simulink model "heli_quanser_base_D"  (R2025a)
settings: Solver=FixedStepAuto  StartTime=0.0  StopTime=30  FixedStep=0.001  RelTol=1e-3  EnableMultiTasking=on
values from neighbouring files (symbols this model uses):
  Ts = 1    [heli_ls_ident.m]    (also in minimos_cuadrados.m)
undefined symbols (not defined in the file or in its folder): B_p, B_y, g, J_eq_p, J_eq_y, K_pp, K_py, K_yp, K_yy, l_cm, m_heli, theta_0, VMAX_UPM_P, VMAX_UPM_Y
libraries: simulink x2, simulink_extras x1
settings Model: Creator=Jorge Romero  LastModifiedBy=Salvador
settings SolverCC: AlgebraicLoopSolver=TrustRegion
settings DataIOCC: LimitDataPoints=on  SaveFormat=Array  ReturnWorkspaceOutputs=off
settings OptimizationCC: ExpressionDepthLimit=2147483647.0  LifeSpan=inf
settings DebuggingCC: UnderspecifiedInitializationDetection=Classic  MergeDetectMultiDrivingBlocksExec=none  SolverPrmCheckMsg=warning  UnconnectedInputMsg=warning  UnconnectedOutputMsg=warning  UnconnectedLineMsg=warning  StateNameClashWarn=warning  SFUnexpectedBacktrackingDiag=warning  SFNoUnconditionalDefaultTransitionDiag=warning  SFExecutionAtInitializationDiag=none  ArithmeticOperatorsInVariantConditions=warning
settings HardwareCC: ProdBitPerPointer=32.0  ProdBitPerSizeT=32.0  ProdBitPerPtrDiffT=32.0  ProdLargestAtomicFloat=None  ProdIntDivRoundTo=Undefined  ProdEndianess=Unspecified  ProdWordSize=32.0  ProdHWDeviceType=32-bit Generic
settings ModelReferenceCC: EnableRefExpFcnMdlSchedulingChecks=on  PropagateSignalLabelsOutOfModel=off
settings SFSimCC: SimUseLocalCustomCode=off  CustomCodeUndefinedFunction=UseInterfaceOnly
settings RTWCC: RTWUseLocalCustomCode=off  GPUComputeCapability=3.5  DLArmComputeVersion=19.05
settings CodeAppCC: StateflowObjectComments=on
settings GRTTargetCC: TargetLangStandard=C89/C90 (ANSI)
settings ConfigComp: CovMetricSettings=dw  CovSaveCumulativeToWorkspaceVar=on  CovSaveSingleToWorkspaceVar=on  CovExternalEMLEnable=off

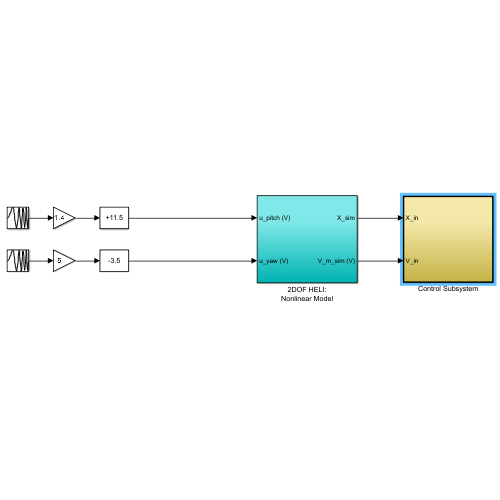
[thumbnail: Simulink's stored preview of the top-level diagram]
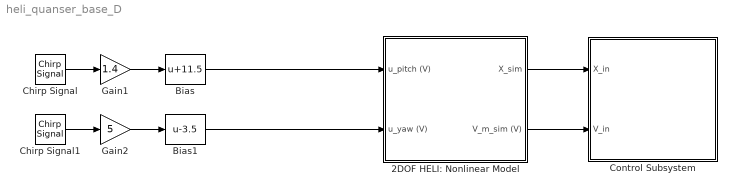
== system heli_quanser_base_D ==
  2DOF HELI: Nonlinear Model : Subsystem
  Bias : Bias  Bias=11.5  SaturateOnIntegerOverflow=off
  Bias1 : Bias  Bias=-3.5  SaturateOnIntegerOverflow=off
  Chirp Signal : simulink/Sources/Chirp Signal  f1=0.08  T=10  f2=1
  Chirp Signal1 : simulink/Sources/Chirp Signal  f1=0.05  T=100  f2=1
  Control Subsystem : Subsystem  TreatAsAtomicUnit=on
  Gain1 : Gain  Gain=1.4
  Gain2 : Gain  Gain=5
  wires:
  Gain2/1 -> Bias1/1
  Gain1/1 -> Bias/1
  Chirp Signal1/1 -> Gain2/1
  Chirp Signal/1 -> Gain1/1
  Bias/1 -> 2DOF HELI: Nonlinear Model/1(u_pitch (V))
  Bias1/1 -> 2DOF HELI: Nonlinear Model/2(u_yaw (V))
  2DOF HELI: Nonlinear Model/1(X_sim) -> Control Subsystem/1(X_in)
  2DOF HELI: Nonlinear Model/2(V_m_sim (V)) -> Control Subsystem/2(V_in)

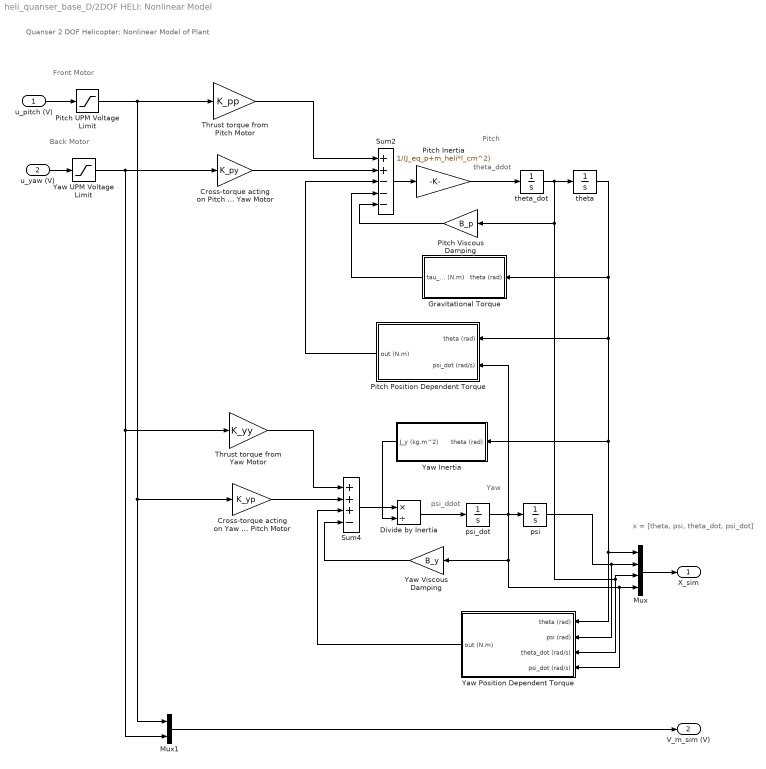
== system heli_quanser_base_D/2DOF HELI: Nonlinear Model ==
  note: Back Motor
  note: Front Motor
  note: x = [theta, psi, theta_dot, psi_dot]
  note: Quanser 2 DOF Helicopter: Nonlinear Model of Plant
  note: theta_ddot
  note: psi_ddot
  note: Pitch
  note: Yaw
  u_pitch (V) : Inport
  u_yaw (V) : Inport  Port=2
  Cross-torque acting on Pitch from Yaw Motor : Gain  Gain=K_py
  Cross-torque acting on Yaw from Pitch Motor : Gain  Gain=K_yp
  Divide by Inertia : Product  Inputs=*/
  Gravitational Torque : Subsystem
  Mux : Mux
  Mux1 : Mux  Inputs=2
  Pitch Inertia : Gain  Gain=1/(J_eq_p+m_heli*l_cm^2)
  Pitch Position Dependent Torque : Subsystem  AncestorBlock=heli_2d_lib/2DOF Helicopter: Nonlinear Model/Yaw Nonlinear Element
  Pitch UPM Voltage Limit : Saturate  UpperLimit=VMAX_UPM_P  LowerLimit=- VMAX_UPM_P
  Pitch Viscous Damping : Gain  Gain=B_p
  Sum2 : Sum  Inputs=++---
  Sum4 : Sum  Inputs=+++-
  Thrust torque from Pitch Motor : Gain  Gain=K_pp
  Thrust torque from Yaw Motor : Gain  Gain=K_yy
  Yaw Inertia : Subsystem
  Yaw Position Dependent Torque : Subsystem
  Yaw UPM Voltage Limit : Saturate  UpperLimit=VMAX_UPM_Y  LowerLimit=- VMAX_UPM_Y
  Yaw Viscous Damping : Gain  Gain=B_y
  psi : Integrator
  psi_dot : Integrator
  theta : Integrator  InitialCondition=theta_0  LimitOutput=on  UpperSaturationLimit=40.5*pi/180  LowerSaturationLimit=-40.5*pi/180
  theta_dot : Integrator
  X_sim : Outport
  V_m_sim (V) : Outport  Port=2
  wires:
  Pitch Position Dependent Torque/1(out (N.m)) -> Sum2/3
  Gravitational Torque/1(tau_g (N.m)) -> Sum2/4
  Pitch Viscous Damping/1 -> Sum2/5
  Cross-torque acting on Pitch from Yaw Motor/1 -> Sum2/2
  Thrust torque from Pitch Motor/1 -> Sum2/1
  Yaw Inertia/1(J_y (kg.m^2)) -> Divide by Inertia/2
  Divide by Inertia/1 -> psi_dot/1
  Sum4/1 -> Divide by Inertia/1
  Yaw Position Dependent Torque/1(out (N.m)) -> Sum4/3
  Yaw Viscous Damping/1 -> Sum4/4
  psi/1 -> Yaw Position Dependent Torque/2(psi (rad)), Mux/2
  Mux1/1 -> V_m_sim (V)/1
  Yaw UPM Voltage Limit/1 -> Thrust torque from Yaw Motor/1, Mux1/2, Cross-torque acting on Pitch from Yaw Motor/1
  Pitch UPM Voltage Limit/1 -> Mux1/1, Cross-torque acting on Yaw from Pitch Motor/1, Thrust torque from Pitch Motor/1
  Mux/1 -> X_sim/1
  theta/1 -> Gravitational Torque/1(theta (rad)), Pitch Position Dependent Torque/1(theta (rad)), Yaw Position Dependent Torque/1(theta (rad)), Mux/1, Yaw Inertia/1(theta (rad))
  Sum2/1 -> Pitch Inertia/1
  Pitch Inertia/1 -> theta_dot/1
  theta_dot/1 -> Pitch Viscous Damping/1, Yaw Position Dependent Torque/3(theta_dot (rad/s)), Mux/3, theta/1
  Thrust torque from Yaw Motor/1 -> Sum4/1
  Cross-torque acting on Yaw from Pitch Motor/1 -> Sum4/2
  psi_dot/1 -> Yaw Viscous Damping/1, Yaw Position Dependent Torque/4(psi_dot (rad/s)), Mux/4, Pitch Position Dependent Torque/2(psi_dot (rad/s)), psi/1
  u_pitch (V)/1 -> Pitch UPM Voltage Limit/1
  u_yaw (V)/1 -> Yaw UPM Voltage Limit/1

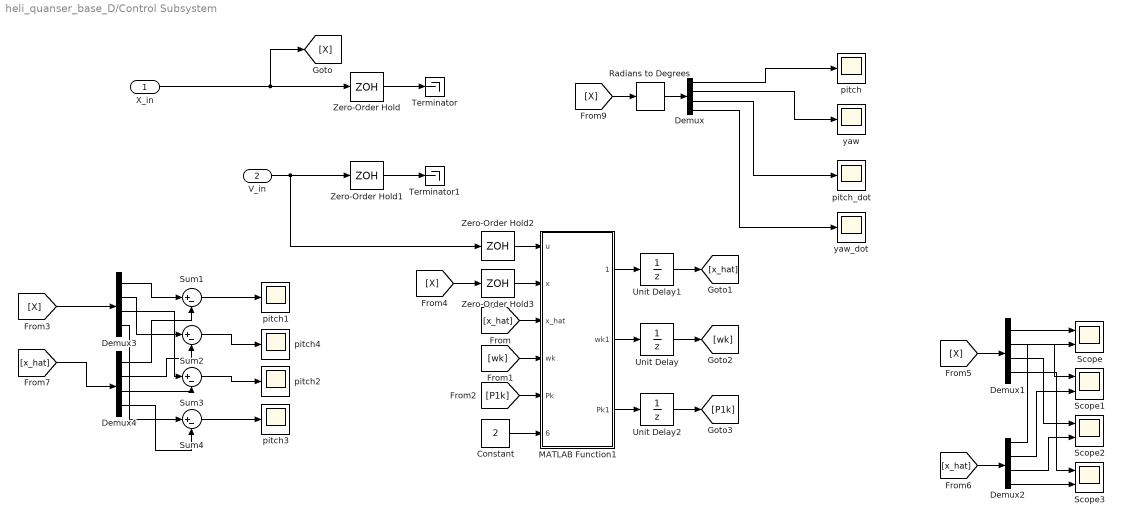
== system heli_quanser_base_D/Control Subsystem ==
  X_in : Inport
  V_in : Inport  Port=2
  Constant : Constant  Value=2
  Demux{,1..4} (5 alike) : Demux
      Demux settings: DisplayOption=none
  MATLAB Function1 : MATLAB Function  TreatAsAtomicUnit=on
  Radians to Degrees : simulink_extras/Transformations/Radians to Degrees
  Scope{,1..3} (4 alike) : Scope  NumInputPorts=2
      Scope settings: ActiveDisplayYMinimum=-0.52190206822218621  ActiveDisplayYMaximum=-0.317262453941132  DataLoggingVariableName=ScopeData4
      Scope1 settings: ActiveDisplayYMinimum=0.00065987107501674913  ActiveDisplayYMaximum=4.6512841717291593  DataLoggingVariableName=ScopeData5
      Scope2 settings: ActiveDisplayYMinimum=-136.21614176214669  ActiveDisplayYMaximum=1171.9792706431781  DataLoggingVariableName=ScopeData6
      Scope3 settings: ActiveDisplayYMinimum=-9.7315281651989078  ActiveDisplayYMaximum=36.666032620078838  DataLoggingVariableName=ScopeData7
  Sum{1..4} (4 alike) : Sum  Inputs=|+-
  Terminator : Terminator
  Terminator1 : Terminator
  Unit Delay : UnitDelay  InitialCondition=rand(16,1)  SampleTime=-1  HasFrameUpgradeWarning=on
  Unit Delay1 : UnitDelay  SampleTime=-1  HasFrameUpgradeWarning=on
  Unit Delay2 : UnitDelay  InitialCondition=repmat(5e4*eye(4), [1 1 4])  SampleTime=-1  HasFrameUpgradeWarning=on
  Zero-Order Hold2 : ZeroOrderHold  SampleTime=-1
  Zero-Order Hold3 : ZeroOrderHold  SampleTime=-1
  Zero-Order Hold : ZeroOrderHold  SampleTime=Ts
  Zero-Order Hold1 : ZeroOrderHold  SampleTime=Ts
  pitch{,1..4} (5 alike) : Scope
      pitch settings: TimeSpan=30  ActiveDisplayYMinimum=-81.99762  ActiveDisplayYMaximum=9.11085
      pitch1 settings: TimeSpan=30  ActiveDisplayYMinimum=-81.99762  ActiveDisplayYMaximum=9.11085  DataLoggingVariableName=ScopeData8
      pitch2 settings: TimeSpan=30  ActiveDisplayYMinimum=-81.99762  ActiveDisplayYMaximum=9.11085  DataLoggingVariableName=ScopeData9
      pitch3 settings: TimeSpan=30  ActiveDisplayYMinimum=-81.99762  ActiveDisplayYMaximum=9.11085  DataLoggingVariableName=ScopeData10
      pitch4 settings: TimeSpan=30  ActiveDisplayYMinimum=-81.99762  ActiveDisplayYMaximum=9.11085  DataLoggingVariableName=ScopeData11
  pitch_dot : Scope
      settings: TimeSpan=30  ActiveDisplayYMinimum=-48.65452  ActiveDisplayYMaximum=62.46494
  yaw : Scope
      settings: TimeSpan=30  ActiveDisplayYMinimum=-31.83031  ActiveDisplayYMaximum=286.47281  DataLoggingVariableName=ScopeData2
  yaw_dot : Scope
      settings: TimeSpan=30  ActiveDisplayYMinimum=-83.27416  ActiveDisplayYMaximum=83.72639  DataLoggingVariableName=ScopeData3
  wires:
  Demux/1 -> pitch/1
  Demux/4 -> yaw_dot/1
  Radians to Degrees/1 -> Demux/1
  [X] -> Radians to Degrees/1
  Demux/3 -> pitch_dot/1
  Demux/2 -> yaw/1
  Zero-Order Hold/1 -> Terminator/1
  Zero-Order Hold1/1 -> Terminator1/1
  [x_hat] -> MATLAB Function1/3(x_hat)
  Unit Delay1/1 -> [x_hat]
  MATLAB Function1/2(wk1) -> Unit Delay/1
  MATLAB Function1/3(Pk1) -> Unit Delay2/1
  Zero-Order Hold2/1 -> MATLAB Function1/1(u)
  Unit Delay2/1 -> [P1k]
  [P1k] -> MATLAB Function1/5(Pk)
  Unit Delay/1 -> [wk]
  MATLAB Function1/1(x_hat_k1) -> Unit Delay1/1
  Zero-Order Hold3/1 -> MATLAB Function1/2(x)
  [wk] -> MATLAB Function1/4(wk)
  V_in/1 -> Zero-Order Hold2/1, Zero-Order Hold1/1
  [X] -> Zero-Order Hold3/1
  Demux1/3 -> Scope2/1
  Demux1/2 -> Scope1/1
  [x_hat] -> Demux2/1
  Demux2/2 -> Scope1/2
  Demux2/4 -> Scope3/2
  Demux2/1 -> Scope/2
  [X] -> Demux1/1
  Demux1/1 -> Scope/1
  Demux1/4 -> Scope3/1
  Demux2/3 -> Scope2/2
  X_in/1 -> [X], Zero-Order Hold/1
  Constant/1 -> MATLAB Function1/6(basis_id)
  Demux3/1 -> Sum1/1
  Demux4/1 -> Sum1/2
  Sum1/1 -> pitch1/1
  Demux3/2 -> Sum2/1
  Demux4/2 -> Sum2/2
  Demux3/3 -> Sum3/1
  Demux4/3 -> Sum3/2
  Demux3/4 -> Sum4/1
  Demux4/4 -> Sum4/2
  Sum4/1 -> pitch3/1
  Sum3/1 -> pitch2/1
  Sum2/1 -> pitch4/1
  [X] -> Demux3/1
  [x_hat] -> Demux4/1

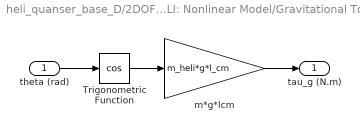
== system heli_quanser_base_D/2DOF HELI: Nonlinear Model/Gravitational Torque ==
  theta (rad) : Inport
  Trigonometric Function : Trigonometry  Operator=cos  OutputSignalType=real
  m*g*lcm : Gain  Gain=m_heli*g*l_cm
  tau_g (N.m) : Outport
  wires:
  m*g*lcm/1 -> tau_g (N.m)/1
  theta (rad)/1 -> Trigonometric Function/1
  Trigonometric Function/1 -> m*g*lcm/1

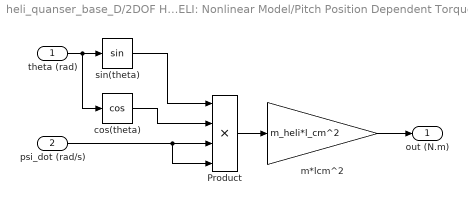
== system heli_quanser_base_D/2DOF HELI: Nonlinear Model/Pitch Position Dependent Torque ==
  theta (rad) : Inport
  psi_dot (rad/s) : Inport  Port=2
  Product : Product  Inputs=4  RndMeth=Zero
  cos(theta) : Trigonometry  Operator=cos  OutputSignalType=real
  m*lcm^2 : Gain  Gain=m_heli*l_cm^2
  sin(theta) : Trigonometry  OutputSignalType=real
  out (N.m) : Outport
  wires:
  psi_dot (rad/s)/1 -> Product/4, Product/3
  theta (rad)/1 -> cos(theta)/1, sin(theta)/1
  Product/1 -> m*lcm^2/1
  sin(theta)/1 -> Product/1
  cos(theta)/1 -> Product/2
  m*lcm^2/1 -> out (N.m)/1

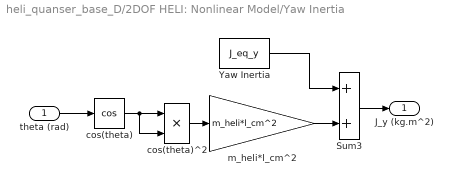
== system heli_quanser_base_D/2DOF HELI: Nonlinear Model/Yaw Inertia ==
  theta (rad) : Inport
  Sum3 : Sum
  Yaw Inertia : Constant  Value=J_eq_y
  cos(theta) : Trigonometry  Operator=cos  OutputSignalType=real
  cos(theta)^2 : Product  RndMeth=Zero
  m_heli*l_cm^2 : Gain  Gain=m_heli*l_cm^2
  J_y (kg.m^2) : Outport
  wires:
  cos(theta)/1 -> cos(theta)^2/2, cos(theta)^2/1
  Sum3/1 -> J_y (kg.m^2)/1
  theta (rad)/1 -> cos(theta)/1
  m_heli*l_cm^2/1 -> Sum3/2
  Yaw Inertia/1 -> Sum3/1
  cos(theta)^2/1 -> m_heli*l_cm^2/1

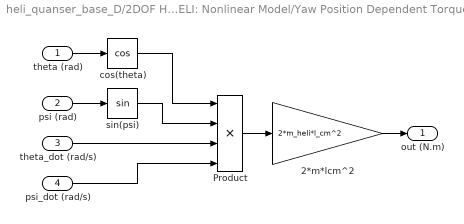
== system heli_quanser_base_D/2DOF HELI: Nonlinear Model/Yaw Position Dependent Torque ==
  theta (rad) : Inport
  psi (rad) : Inport  Port=2
  theta_dot (rad/s) : Inport  Port=3
  psi_dot (rad/s) : Inport  Port=4
  2*m*lcm^2 : Gain  Gain=2*m_heli*l_cm^2
  Product : Product  Inputs=4  RndMeth=Zero
  cos(theta) : Trigonometry  Operator=cos  OutputSignalType=real
  sin(psi) : Trigonometry  OutputSignalType=real
  out (N.m) : Outport
  wires:
  2*m*lcm^2/1 -> out (N.m)/1
  psi_dot (rad/s)/1 -> Product/4
  theta_dot (rad/s)/1 -> Product/3
  sin(psi)/1 -> Product/2
  cos(theta)/1 -> Product/1
  Product/1 -> 2*m*lcm^2/1
  theta (rad)/1 -> cos(theta)/1
  psi (rad)/1 -> sin(psi)/1

== matlab function heli_quanser_base_D/Control Subsystem/MATLAB Function1 ==
  data: u input; x input; x_hat input; wk input; Pk input; x_hat_k1 output; wk1 output; Pk1 output; basis_id input
function [x_hat_k1, wk1, Pk1] = rhonn_rotary(u, x, x_hat, wk, Pk, basis_id)
% RHONN para péndulo rotatorio (Furuta) con 4 estados:
% x = [beta; betadot; gamma; gammadot]
%
% basis_id: entero
%   1=tanh, 2=sigmoid, 3=relu, 4=leakyrelu, 5=sin, 6=poly2,
%   7=elu, 8=swish, 9=rbf

%% Defaults
if nargin < 7, basis_id = 1; end  % tanh default
alpha = 0.01;        % usado por leakyrelu/elu/swish
Q = eye(4)*5e3;
R = 6e3;
w_u2 = [0.15; 0.00];
w_u4 = [0.00; 0.15];
rbf_c = zeros(4,1);
rbf_s = ones(4,1);

%% Regresores no lineales (H = phi(x))
a = alpha;
switch basis_id
    case 1   % tanh
        H = tanh(x);
    case 2   % sigmoid
        H = 1./(1+exp(-x));
    case 3   % relu
        H = max(0, x);
    case 4   % leakyrelu
        H = max(x, a*x);
    case 5   % sin
        H = sin(a*x);
    case 6   % poly2
        H = x.^2;
    case 7   % elu
        H = x;
        m = x<0; H(m) = a*(exp(x(m))-1);
    case 8   % swish
        H = x .* (1./(1+exp(-a*x)));
    case 9   % rbf
        s = rbf_s; s(s<=0)=1;
        H = exp(-0.5 * ((x - rbf_c)./s).^2);
    otherwise
        H = tanh(x);   % fallback seguro
end

%% Extraer pesos
w1 = wk(1:4); w2 = wk(5:8); w3 = wk(9:12); w4 = wk(13:16);

%% Predicción neuronal
x1_hat = w1.'*H;
x2_hat = w2.'*H + w_u2.'*u;
x3_hat = w3.'*H;
x4_hat = w4.'*H + w_u4.'*u;
x_hat_k1 = [x1_hat; x2_hat; x3_hat; x4_hat];

%% EKF por estado
Pk1 = Pk; wk1 = wk;
e = x - x_hat;

for i = 1:4
    Pi = Pk(:,:,i);
    Ki = (Pi*H)/(R + H.'*Pi*H);
    wi = wk((i-1)*4+1:i*4);
    wi_new = wi + Ki*e(i);
    Pi_new = Pi - Ki*(H.')*Pi + Q;
    wk1((i-1)*4+1:i*4) = wi_new;
    Pk1(:,:,i) = Pi_new;
end

end
